simulink model "motor_model_v2_failed"  (R2016a)
settings: Solver=VariableStepAuto  StartTime=0.0  StopTime=1  RelTol=1e-3
settings Model: Creator=user  LastModifiedBy=user

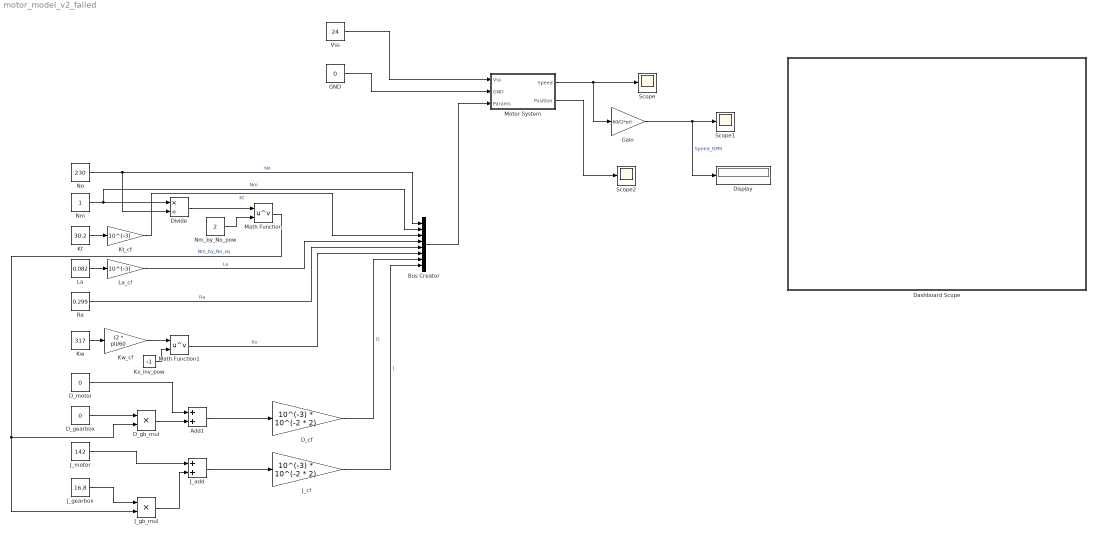
== system motor_model_v2_failed ==
  Add1 : Sum
  Bus Creator : BusCreator  Inputs=8
  D_cf : Gain  Gain=10^(-3) * 10^(-2 * 2)
  D_gb_mul : Product  Inputs=**
  D_gearbox : Constant  Value=0
  D_motor : Constant  Value=0
  Dashboard Scope : Subsystem  DialogController=hmiCreateDDGDialog  IsWebBlock=on  mask(MWDashboardBlock){webBlockId=ecdd70a7-2b72-4acf-bca9-833aaf066668, webBlockType=sdiscope, ShowInitialText=on, HMISrcModelName=motor_model_v2}
      mask prompts: webBlockId "WebBlock Id"; webBlockType "WebBlock Type"; HMISrcModelName "Source Model"
      mask Help: helpview([docroot '/mapfiles/simulink.map'], 'hmi_scope')
      mask Display:
      | if strcmp(get_param(bdroot(gcb),'BlockDiagramType'), 'library')
      |     image([(matlabroot) '/toolbox/simulink/hmi/icons/DashboardScope.png']);
      | end
  Display : Display
      settings: Decimation=4
  Divide : Product  Inputs=*/
  GND : Constant  Value=0
  Gain : Gain  Gain=60/(2*pi)
  J_add : Sum
  J_cf : Gain  Gain=10^(-3) * 10^(-2 * 2)
  J_gb_mul : Product  Inputs=**
  J_gearbox : Constant  Value=16.8
  J_motor : Constant  Value=142
  Kt : Constant  Value=30.2
  Kt_cf : Gain  Gain=10^(-3)
  Kv_inv_pow : Constant  Value=-1
  Kw : Constant  Value=317
  Kw_cf : Gain  Gain=(2 * pi)/60
  La : Constant  Value=0.082
  La_cf : Gain  Gain=10^(-3)
  Math Function : Math  Operator=pow  SaturateOnIntegerOverflow=on
  Math Function1 : Math  Operator=pow  SaturateOnIntegerOverflow=on
  Motor System : Subsystem
  Nm : Constant
  Nm_by_No_pow : Constant  Value=2
  No : Constant  Value=230
  Ra : Constant  Value=0.299
  Scope : Scope
  Scope1 : Scope
  Scope2 : Scope
  Vss : Constant  Value=24
  wires:
  Vss/1 -> Motor System/1(Vss)
  GND/1 -> Motor System/2(GND)
  Motor System/1(Speed) -> Gain/1, Scope/1
  Gain/1 -> Display/1, Scope1/1  "Speed_RPM"
  Motor System/2(Position) -> Scope2/1
  Kt/1 -> Kt_cf/1
  La/1 -> La_cf/1
  Kw/1 -> Kw_cf/1
  Nm/1 -> Bus Creator/2, Divide/1  "Nm"
  No/1 -> Divide/2, Bus Creator/1  "No"
  Nm_by_No_pow/1 -> Math Function/2
  Divide/1 -> Math Function/1
  Math Function/1 -> D_gb_mul/2, J_gb_mul/2  "Nm_by_No_sq"
  J_gearbox/1 -> J_gb_mul/1
  J_gb_mul/1 -> J_add/2
  J_motor/1 -> J_add/1
  J_add/1 -> J_cf/1
  Kt_cf/1 -> Bus Creator/3  "Kt"
  La_cf/1 -> Bus Creator/4  "La"
  Ra/1 -> Bus Creator/5  "Ra"
  Kw_cf/1 -> Math Function1/1
  Kv_inv_pow/1 -> Math Function1/2
  Math Function1/1 -> Bus Creator/6  "Kv"
  D_gearbox/1 -> D_gb_mul/1
  D_motor/1 -> Add1/1
  D_gb_mul/1 -> Add1/2
  Add1/1 -> D_cf/1
  D_cf/1 -> Bus Creator/7  "D"
  J_cf/1 -> Bus Creator/8  "J"
  Bus Creator/1 -> Motor System/3(Params)

== system motor_model_v2_failed/Dashboard Scope ==

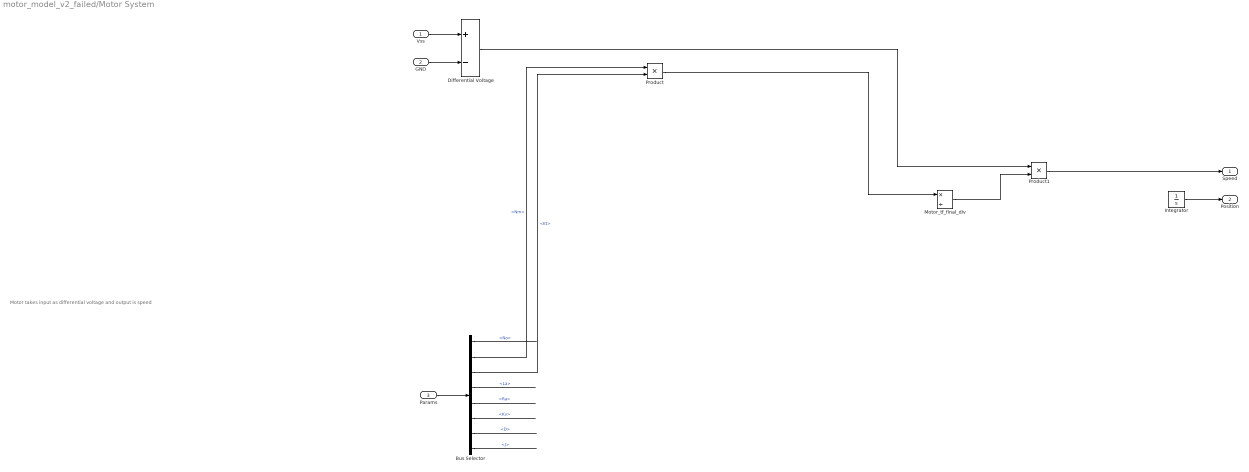
== system motor_model_v2_failed/Motor System ==
  note: Motor takes input as differential voltage and output is speed
  Vss : Inport
  GND : Inport  Port=2
  Params : Inport  Port=3
  Bus Selector : BusSelector  OutputSignals=No,Nm,Kt,La,Ra,Kv,D,J
  Differential Voltage : Sum  Inputs=+-
  Integrator : Integrator
  Motor_tf_final_div : Product  Inputs=*/
  Product : Product
  Product1 : Product
  Speed : Outport
  Position : Outport  Port=2
  wires:
  Vss/1 -> Differential Voltage/1
  GND/1 -> Differential Voltage/2
  Integrator/1 -> Position/1
  Params/1 -> Bus Selector/1
  Bus Selector/1 -> ?  "<No>"
  Bus Selector/2 -> Product/1  "<Nm>"
  Bus Selector/3 -> Product/2  "<Kt>"
  Bus Selector/4 -> ?  "<La>"
  Bus Selector/5 -> ?  "<Ra>"
  Bus Selector/6 -> ?  "<Kv>"
  Bus Selector/7 -> ?  "<D>"
  Bus Selector/8 -> ?  "<J>"
  Product/1 -> Motor_tf_final_div/1
  Product1/1 -> Speed/1
  Motor_tf_final_div/1 -> Product1/2
  Differential Voltage/1 -> Product1/1
